simulink model "Perturb_and_Observe_Algorithm"  (R2017b)
settings: Solver=VariableStepDiscrete  StartTime=0.0  StopTime=10  MaxStep=1e-3  RelTol=1e-3
undefined symbols (not defined in the file): Acid, Down, Lead, sigbuilder_block, Up
libraries: powerlib x33, electricdrivelib x1, re_lib x1, pePwmGenerator x1
settings Model: Creator=NGBNTA001  LastModifiedBy=NGBNTA001
settings SolverCC: ZeroCrossAlgorithm=Adaptive
settings DebuggingCC: IgnoredZcDiagnostic=none

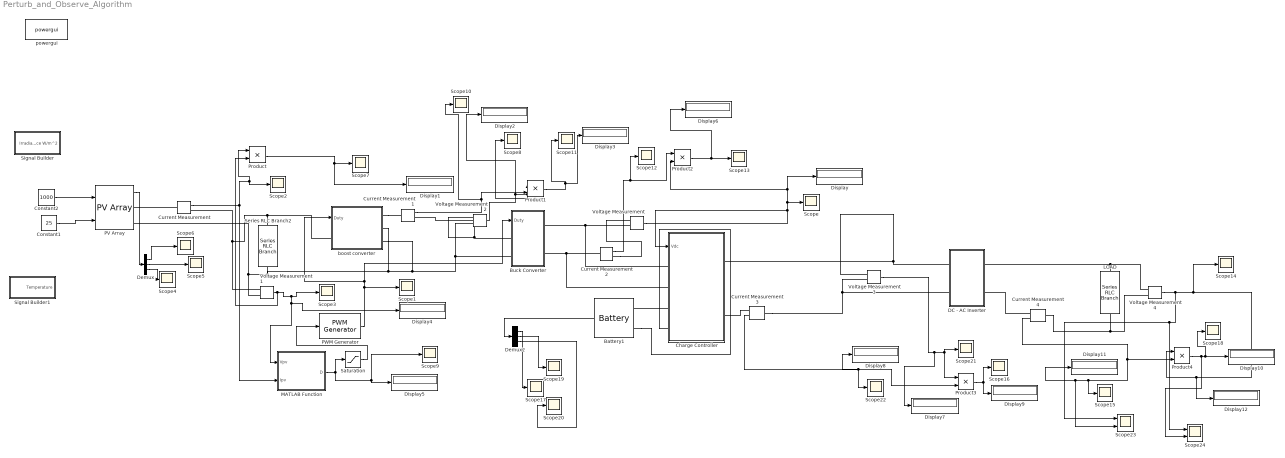
== system Perturb_and_Observe_Algorithm ==
  Battery1 : electricdrivelib/Extra Sources/Battery  BatType=Lead-Acid  ShowTempParam=off  ThermalPreset=no  ShowAgeParam=off  NomV=230  NomQ=240  SOC=50  Batt_Tr=30  PresetModel=on  MaxQ=250  MinV=172.5  FullV=250.4276  Dis_rate=48  R=0.0095833  Normal_OP=74.4667  expZone="[234.1612           0.8]"  current=[10 29.18 64.7]  Units=Time  Tci=20  NomT=20  T2=-30  MaxQ2=4.8  FullV2=7.1  Normal_OP2=5.655  expZone2="[6.58           1]"  Rca=0.6  ti=2000  Dp=0  Neq0=0  Tsim=1e6  Ta1=25  Qeol=5.4*0.9  Reol=0.013333*1.2  Char_age=[2.3478, 3]  Dis_age=[2.3478, 10]  N1=1500  N2=10500  N3=1000  N4=1400  Ta2=45  N5=950
  Buck Converter : Subsystem
  Charge Controller : Subsystem
  Constant1 : Constant  Value=25
  Constant2 : Constant  Value=1000
  Current Measurement{,1..4} (5 alike) : powerlib/Measurements/Current Measurement  PhasorSimulation=off  OutputType=Complex  PSBequivalent=0
  DC - AC Inverter : Subsystem
  Demux : Demux  Outputs=3
  Demux2 : Demux  Outputs=3
  Display{,1..12} (13 alike) : Display
  LOAD : powerlib/Elements/Series RLC Branch  LConnTagsString=__new0  RConnTagsString=__new0  BranchType=R  Resistance=7.84  Inductance=1e-3  SetiL0=off  InitialCurrent=0  Capacitance=1e-6  Setx0=off  InitialVoltage=0  Measurements=None
  MATLAB Function : MATLAB Function  TreatAsAtomicUnit=on  SystemSampleTime=0.01
  PV Array : re_lib/Solar/PV Array  Npar=2  Nser=15  PlotType=array @ 1000 W/m2 & specified temperatures  S_vec="[ 1000  800  600 400 200 0 ]"  Temp_C_vec="[ 40 25 10 0  ]"  ModuleName=1Soltech 1STH-215-P  PlotWhenSelected=off  Pm=213.15  Ncell=60  Voc=36.3  Isc=7.84  Vm=29  Im=7.35  beta_Voc_pc=-0.36099  alpha_Isc_pc=0.102  beta_Voc=-0.13104  alpha_Isc=0.007997  IL=7.8649  I0=2.9259e-10  nI=0.98117  Rsh=313.3991  Rs=0.39383  BAL=off  Tc=1e-6  Tfilter=0.001
  PWM Generator : pePwmGenerator/PWM Generator  CarrCount=Up-Down  Tper=0.001  Ts=5e-6
  Product{,1..4} (5 alike) : Product
  Saturation : Saturate  UpperLimit=1  LowerLimit=0
  Scope{,1..22} (23 alike) : Scope
  Scope23 : Scope  NumInputPorts=2
  Scope24 : Scope  NumInputPorts=2
  Series RLC Branch2 : powerlib/Elements/Series RLC Branch  LConnTagsString=__new0  RConnTagsString=__new0  BranchType=C  Resistance=1  Inductance=47e-3  SetiL0=off  InitialCurrent=0  Capacitance=470e-6  Setx0=off  InitialVoltage=0  Measurements=None
  Signal Builder : Subsystem  Tag=STV Subsys  LoadFcn=sigbuilder_block('load');  StartFcn=sigbuilder_block('start');  StopFcn=sigbuilder_block('stop');  ClipboardFcn=sigbuilder_block('clipboard');  mask(Sigbuilder block){tuvar=[0:10]}
      mask help: Simulink:masks:SigbuilderBlock_MD
      mask init:
      | if ~strcmp(get_param(bdroot(gcbh),'SimulationStatus'),'stopped') tuvar = sigbuilder_block('maskInit'); end
      settings: CopyFcn=sigbuilder_block('copy');  DeleteFcn=sigbuilder_block('delete');  ModelCloseFcn=sigbuilder_block('modelClose');  PreSaveFcn=sigbuilder_block('preSave');  PauseFcn=sigbuilder_block('pause');  ContinueFcn=sigbuilder_block('continue');  NameChangeFcn=sigbuilder_block('namechange');  OpenFcn=sigbuilder_block('open',[6 30 1428 681.75 ]);  CloseFcn=sigbuilder_block('close');
      mask Display: plot(0, 0, 100, 100,[2, 2, 32, 32, 2], [68, 8, 8, 68, 68],[32, 2], [38, 38], [32, 19, 2],[53, 60, 44], [32, 17, 17, 2],[16, 16, 31, 31]);txt = getActiveGroup(gcbh);text(2, 100, txt,'verticalAlignment', 'top');
  Signal Builder1 : Subsystem  Tag=STV Subsys  LoadFcn=sigbuilder_block('load');  StartFcn=sigbuilder_block('start');  StopFcn=sigbuilder_block('stop');  ClipboardFcn=sigbuilder_block('clipboard');  mask(Sigbuilder block){tuvar=[0:10]}
      mask help: Simulink:masks:SigbuilderBlock_MD
      mask init:
      | if ~strcmp(get_param(bdroot(gcbh),'SimulationStatus'),'stopped') tuvar = sigbuilder_block('maskInit'); end
      settings: CopyFcn=sigbuilder_block('copy');  DeleteFcn=sigbuilder_block('delete');  ModelCloseFcn=sigbuilder_block('modelClose');  PreSaveFcn=sigbuilder_block('preSave');  PauseFcn=sigbuilder_block('pause');  ContinueFcn=sigbuilder_block('continue');  NameChangeFcn=sigbuilder_block('namechange');  OpenFcn=sigbuilder_block('open',[6 30 1428 681.75 ]);  CloseFcn=sigbuilder_block('close');
      mask Display: plot(0, 0, 100, 100,[2, 2, 32, 32, 2], [68, 8, 8, 68, 68],[32, 2], [38, 38], [32, 19, 2],[53, 60, 44], [32, 17, 17, 2],[16, 16, 31, 31]);txt = getActiveGroup(gcbh);text(2, 100, txt,'verticalAlignment', 'top');
  Voltage Measurement{,1..4} (5 alike) : powerlib/Measurements/Voltage Measurement  PhasorSimulation=off  OutputType=Complex  PSBequivalent=0
  boost converter : Subsystem
  powergui : powerlib/powergui  Priority=1  SimulationMode=Discrete  SampleTime=5e-6  frequency=60  Iterations=50  frequencyindice=0  Pbase=100e6  ErrMax=1e-4  UnitsV=kV  UnitsW=MW  buscounter=0  FunctionMessages=off  echomessages=off  EnableUseOfTLC=off  CurrentSourceSwitches=off  DisableSnubberDevices=off  DisableRonSwitches=off  DisableVfSwitches=off  DisplayEquations=off  SolverType=Tustin/Backward Euler (TBE)  Interpol=off  ExternalGateDelay=off  methode=off  Ts=100  x0status=blocks  SPID=on  SwTol=0  HookPort=off  RestoreLinks=warning  ResistiveCurrentMeasurement=off  Frange=[0:2:500]  Ylog=off  Xlog=on  ShowGrid=off  save=off  variable=ZData  structure=0  ZoomFFT=off  StartTime=0.0  cycles=1  DisplayStyle=1  fundamental=60  FreqAxis=off  MaxFrequency=1000  frequencyindicesteady=1  RmsSteady=1  display=off
  wires:
  Voltage Measurement1/1 -> Product/2, Display4/1, MATLAB Function/1(Vpv), Scope3/1
  Current Measurement/1 -> Product/1, Scope2/1, MATLAB Function/2(Ipv)
  MATLAB Function/1(D) -> Display5/1, Scope9/1, Saturation/1
  PV Array/1 -> Demux/1
  Demux/1 -> Scope6/1
  Demux/2 -> Scope5/1
  Demux/3 -> Scope4/1
  Product/1 -> Display1/1, Scope7/1
  Current Measurement1/1 -> Product1/2, Scope10/1
  Product1/1 -> Display3/1, Scope11/1
  Voltage Measurement2/1 -> Product1/1, Scope8/1, Display2/1
  Saturation/1 -> PWM Generator/1
  PWM Generator/1 -> Buck Converter/1(Duty), boost converter/1(Duty), Scope1/1
  Voltage Measurement/1 -> Display/1, Product2/2, Scope/1, Charge Controller/1(Vdc)
  Current Measurement2/1 -> Product2/1, Scope12/1
  Product2/1 -> Scope13/1, Display6/1
  Demux2/1 -> Scope17/1
  Demux2/2 -> Scope19/1
  Voltage Measurement3/1 -> Scope21/1, Product3/1, Display7/1
  Battery1/1 -> Demux2/1
  Product3/1 -> Display9/1, Scope16/1
  Current Measurement3/1 -> Scope22/1, Product3/2, Display8/1
  Demux2/3 -> Scope20/1
  Voltage Measurement4/1 -> Scope24/1, Scope23/1, Display12/1, Product4/1, Scope14/1
  Current Measurement4/1 -> Scope15/1, Scope23/2, Display11/1, Product4/2
  Product4/1 -> Scope24/2, Scope18/1, Display10/1
  Constant2/1 -> PV Array/1
  Constant1/1 -> PV Array/2
  connections:
  Voltage Measurement2/LConn1 -- Current Measurement1/RConn1 -- Buck Converter/LConn1
  Current Measurement/LConn1 -- PV Array/RConn1
  Voltage Measurement1/LConn1 -- boost converter/LConn1 -- Series RLC Branch2/LConn1 -- Current Measurement/RConn1
  Voltage Measurement1/LConn2 -- PV Array/RConn2 -- Series RLC Branch2/RConn1 -- boost converter/RConn3 -- Buck Converter/LConn2 -- Voltage Measurement2/LConn2 -- boost converter/RConn2
  boost converter/RConn1 -- Current Measurement1/LConn1
  Current Measurement2/RConn1 -- Voltage Measurement/LConn1
  Buck Converter/RConn1 -- Voltage Measurement/LConn2 -- Charge Controller/LConn1
  DC - AC Inverter/LConn2 -- Current Measurement3/LConn1 -- Voltage Measurement3/LConn2
  Voltage Measurement3/LConn1 -- Charge Controller/RConn1 -- DC - AC Inverter/LConn1
  Current Measurement4/LConn1 -- Voltage Measurement4/LConn2 -- LOAD/RConn1
  Current Measurement4/RConn1 -- DC - AC Inverter/RConn2
  Current Measurement2/LConn1 -- Charge Controller/LConn2 -- Buck Converter/RConn2
  Charge Controller/LConn3 -- Battery1/LConn1
  Battery1/LConn2 -- Charge Controller/LConn4
  Current Measurement3/RConn1 -- Charge Controller/RConn2
  Voltage Measurement4/LConn1 -- DC - AC Inverter/RConn1 -- LOAD/LConn1

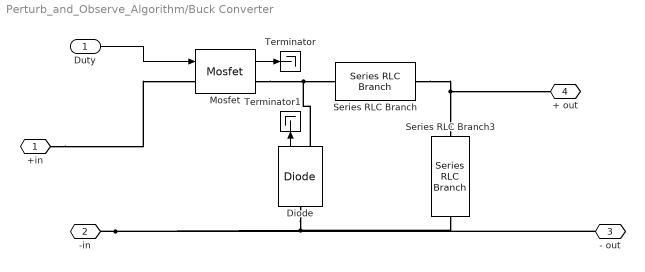
== system Perturb_and_Observe_Algorithm/Buck Converter ==
  Duty : Inport
  Diode : powerlib/Power Electronics/Diode  Ron=0.001  Lon=0  Vf=0.8  IC=0  UseSnubber=0  Rs=500  Cs=250e-9  Measurements=on
  Mosfet : powerlib/Power Electronics/Mosfet  Ron=0.1  Lon=0  Rd=0.01  Vfd=0  IC=0  Rs=1e5  Cs=inf  Measurements=on
  Series RLC Branch : powerlib/Elements/Series RLC Branch  LConnTagsString=__new0  RConnTagsString=__new0  BranchType=L  Resistance=1  Inductance=1e-3  SetiL0=off  InitialCurrent=0  Capacitance=1e-6  Setx0=off  InitialVoltage=0  Measurements=None
  Series RLC Branch3 : powerlib/Elements/Series RLC Branch  LConnTagsString=__new0  RConnTagsString=__new0  BranchType=C  Resistance=1  Inductance=1e-3  SetiL0=off  InitialCurrent=0  Capacitance=470e-6  Setx0=off  InitialVoltage=0  Measurements=None
  Terminator : Terminator
  Terminator1 : Terminator
  +in : PMIOPort  Port=1  Side=Left
  -in : PMIOPort  Port=2  Side=Left
  - out : PMIOPort  Port=3  Side=Right
  + out : PMIOPort  Port=4  Side=Right
  wires:
  Duty/1 -> Mosfet/1
  Diode/1 -> Terminator1/1
  Mosfet/1 -> Terminator/1
  connections:
  +in/RConn1 -- Mosfet/LConn1
  Mosfet/RConn1 -- Diode/RConn1 -- Series RLC Branch/LConn1
  Series RLC Branch/RConn1 -- Series RLC Branch3/LConn1 -- + out/RConn1
  -in/RConn1 -- Diode/LConn1 -- - out/RConn1 -- Series RLC Branch3/RConn1

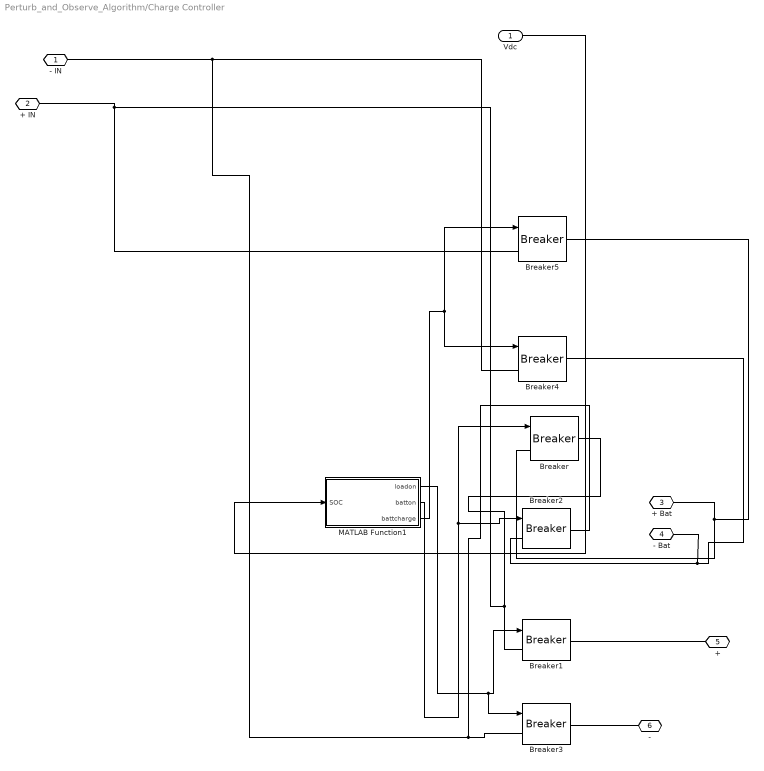
== system Perturb_and_Observe_Algorithm/Charge Controller ==
  Vdc : Inport
  Breaker{,1..5} (6 alike) : powerlib/Elements/Breaker  InitialState=0  SwitchingTimes="[1/60  5/60]"  External=on  BreakerResistance=0.01  SnubberResistance=1e6  SnubberCapacitance=inf  Measurements=None  MoreParameters=on  NoBreakLoop=off
      settings: SourceProductName=Simscape Power Systems
  MATLAB Function1 : MATLAB Function  TreatAsAtomicUnit=on
  - IN : PMIOPort  Port=1  Side=Left
  + IN : PMIOPort  Port=2  Side=Left
  + Bat : PMIOPort  Port=3  Side=Left
  - Bat : PMIOPort  Port=4  Side=Left
  + : PMIOPort  Port=5  Side=Right
  - : PMIOPort  Port=6  Side=Right
  wires:
  Vdc/1 -> MATLAB Function1/1(SOC)
  MATLAB Function1/2(batton) -> Breaker2/1, Breaker/1
  MATLAB Function1/1(loadon) -> Breaker3/1, Breaker1/1
  MATLAB Function1/3(battcharge) -> Breaker5/1, Breaker4/1
  connections:
  Breaker3/LConn1 -- - IN/RConn1 -- Breaker4/LConn1 -- Breaker2/RConn1
  +/RConn1 -- Breaker1/RConn1
  Breaker1/LConn1 -- + IN/RConn1 -- Breaker5/LConn1 -- Breaker/RConn1
  Breaker/LConn1 -- + Bat/RConn1 -- Breaker5/RConn1
  -/RConn1 -- Breaker3/RConn1
  Breaker4/RConn1 -- - Bat/RConn1 -- Breaker2/LConn1

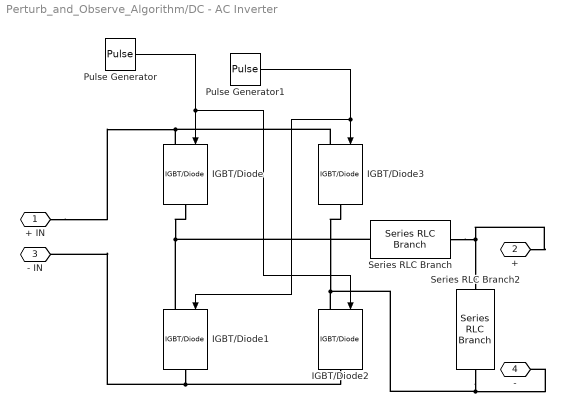
== system Perturb_and_Observe_Algorithm/DC - AC Inverter ==
  IGBT/Diode{,1..3} (4 alike) : powerlib/Power Electronics/IGBT//Diode  Ron=1e-3  Rs=1e5  Cs=inf  Measurements=off
  Pulse Generator : DiscretePulseGenerator  PulseType=Time based  Amplitude=10  Period=1/50  PulseWidth=50
  Pulse Generator1 : DiscretePulseGenerator  PulseType=Time based  Amplitude=10  Period=1/50  PulseWidth=50  PhaseDelay=1/100
  Series RLC Branch : powerlib/Elements/Series RLC Branch  LConnTagsString=__new0  RConnTagsString=__new0  BranchType=L  Resistance=1  Inductance=31e-3  SetiL0=off  InitialCurrent=0  Capacitance=1e-6  Setx0=off  InitialVoltage=0  Measurements=None
  Series RLC Branch2 : powerlib/Elements/Series RLC Branch  LConnTagsString=__new0  RConnTagsString=__new0  BranchType=C  Resistance=1  Inductance=1e-3  SetiL0=off  InitialCurrent=0  Capacitance=470e-6  Setx0=off  InitialVoltage=0  Measurements=None
  + IN : PMIOPort  Port=1  Side=Left
  + : PMIOPort  Port=2  Side=Right
  - IN : PMIOPort  Port=3  Side=Left
  - : PMIOPort  Port=4  Side=Right
  wires:
  Pulse Generator/1 -> IGBT/Diode2/1, IGBT/Diode/1
  Pulse Generator1/1 -> IGBT/Diode3/1, IGBT/Diode1/1
  connections:
  IGBT/Diode3/LConn1 -- IGBT/Diode/LConn1 -- + IN/RConn1
  IGBT/Diode/RConn1 -- Series RLC Branch/LConn1 -- IGBT/Diode1/LConn1
  IGBT/Diode2/RConn1 -- - IN/RConn1 -- IGBT/Diode1/RConn1
  Series RLC Branch2/RConn1 -- IGBT/Diode3/RConn1 -- IGBT/Diode2/LConn1 -- -/RConn1
  Series RLC Branch/RConn1 -- Series RLC Branch2/LConn1 -- +/RConn1

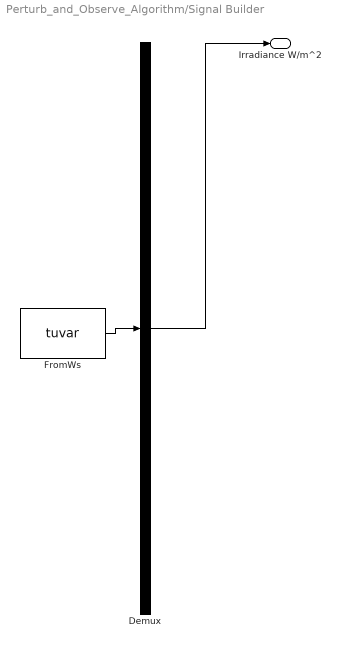
== system Perturb_and_Observe_Algorithm/Signal Builder ==
  Demux : Demux  Tag=STV Demux  Outputs=1
  FromWs : FromWorkspace  Tag=STV FromWs  VariableName=tuvar  SampleTime=0
      SigBuilderData=|
      | common.afterFinalStr = 'Extrapolate'
      | common.sampleTime = 0
      | dataSet.timeRange = [0 10]
      | dataSet.name = 'Group 1'
      | sbobj.Groups.Name = 'Group 1'
      | sbobj.Groups.Signals.Name = 'Irradiance W/m^2'
      | sbobj.Groups.Signals.XData = [0 1 1 2 2 3 3 4 4 5 6 6 7 8 8 9 10]
      | sbobj.Groups.Signals.YData = [0 0 200 200 395 395 396 396 600 600 600 800 800 800 1000 1000 1000]
  Irradiance W/m^2 : Outport  Tag=STV Outport
  wires:
  Demux/1 -> Irradiance W/m^2/1
  FromWs/1 -> Demux/1

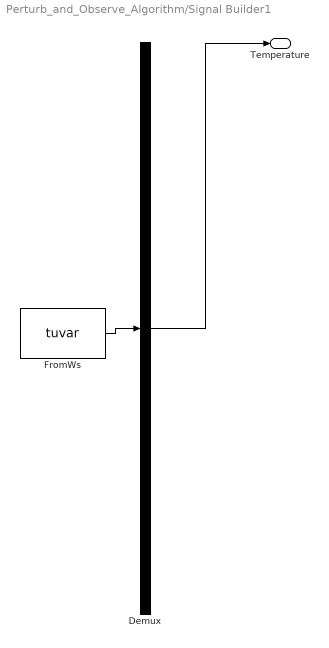
== system Perturb_and_Observe_Algorithm/Signal Builder1 ==
  Demux : Demux  Tag=STV Demux  Outputs=1
  FromWs : FromWorkspace  Tag=STV FromWs  VariableName=tuvar  SampleTime=0
      SigBuilderData=|
      | common.afterFinalStr = 'Extrapolate'
      | common.sampleTime = 0
      | dataSet.timeRange = [0 10]
      | dataSet.name = 'Group 1'
      | sbobj.Groups.Name = 'Group 1'
      | sbobj.Groups.Signals.Name = 'Temperature '
      | sbobj.Groups.Signals.XData = [0 1 2 2 3 3 4 5 6 6 7 8 8 9 10]
      | sbobj.Groups.Signals.YData = [15 15 15 15.05 15.05 25 25 25 25 35 35 35 45 45 45]
  "Temperature " : Outport  Tag=STV Outport
  wires:
  Demux/1 -> "Temperature "/1
  FromWs/1 -> Demux/1

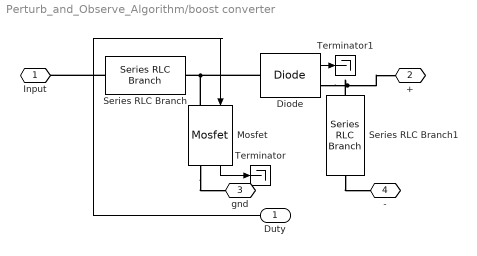
== system Perturb_and_Observe_Algorithm/boost converter ==
  Duty : Inport
  Diode : powerlib/Power Electronics/Diode  Ron=0.001  Lon=0  Vf=0.8  IC=0  UseSnubber=0  Rs=500  Cs=250e-9  Measurements=on
  Mosfet : powerlib/Power Electronics/Mosfet  Ron=0.1  Lon=0  Rd=0.01  Vfd=0  IC=0  Rs=1e5  Cs=inf  Measurements=on
  Series RLC Branch : powerlib/Elements/Series RLC Branch  LConnTagsString=__new0  RConnTagsString=__new0  BranchType=L  Resistance=1  Inductance=10e-3  SetiL0=off  InitialCurrent=0  Capacitance=1e-6  Setx0=off  InitialVoltage=0  Measurements=None
  Series RLC Branch1 : powerlib/Elements/Series RLC Branch  LConnTagsString=__new0  RConnTagsString=__new0  BranchType=C  Resistance=1  Inductance=47e-3  SetiL0=off  InitialCurrent=0  Capacitance=470e-6  Setx0=off  InitialVoltage=0  Measurements=None
  Terminator : Terminator
  Terminator1 : Terminator
  Input : PMIOPort  Port=1  Side=Left
  + : PMIOPort  Port=2  Side=Right
  gnd : PMIOPort  Port=3  Side=Right
  - : PMIOPort  Port=4  Side=Right
  wires:
  Diode/1 -> Terminator1/1
  Duty/1 -> Mosfet/1
  Mosfet/1 -> Terminator/1
  connections:
  Mosfet/RConn1 -- gnd/RConn1
  Series RLC Branch1/RConn1 -- -/RConn1
  Series RLC Branch/LConn1 -- Input/RConn1
  Mosfet/LConn1 -- Diode/LConn1 -- Series RLC Branch/RConn1
  Diode/RConn1 -- +/RConn1 -- Series RLC Branch1/LConn1

== matlab function Perturb_and_Observe_Algorithm/Charge Controller/MATLAB Function1 ==
  data: SOC input; loadon output; batton output; battcharge output
function [loadon,batton,battcharge] = fcn(SOC)
loadon=1;
batton=0;
battcharge=0;
if (SOC>=235)
    loadon=1;
    batton=0;
    battcharge=1;
end
if (SOC<230)
    loadon=1;
    batton=1;
    battcharge=0;
end

== matlab function Perturb_and_Observe_Algorithm/MATLAB Function ==
  data: Vpv input; D output; Ipv input
%This code impliments the Perturb and Observe algorithm.
%it was sourced from EEE world on youtube video and modified. 
%link: https://www.youtube.com/watch?v=6bZla7J4wz0&list=LLwVna-4AQ-FCjOjEW3MMVkw&index=22&t=0s 
function D = TANDO(Vpv,Ipv)
% internal value of voltage
persistent Dprev Pprev Vprev
% initialise values
if isempty(Dprev)
    Dprev=0.6;
    Vprev =100;
    Pprev =200;
end

% initialise algorithm parameters
delD = 0.001;
%Calculate array power
Ppv = Vpv*Ipv;
% conditions for changing duty cycle
if (Ppv-Pprev)~= 0
    if (Ppv-Pprev) > 0
        if (Vpv-Vprev) > 0
            D = Dprev-delD;
        else
            D = Dprev+delD;
        end
    else
        if (Vpv-Vprev)>0
            D = Dprev+delD;
        else 
            D = Dprev-delD;
        end
    end
else
    D= Dprev;
end
Dprev=D;
Vprev =Vpv;
Pprev = Ppv;
